simulink model "export_example"  (Simulink 8.0)
settings: Solver=ode45  StartTime=0.0  StopTime=10.0  RelTol=1e-3
libraries: aerolibactuator x1
settings Model: Creator=Marci  LastModifiedBy=Marci
settings ConfigurationSet: Description=SimMechanics 2G

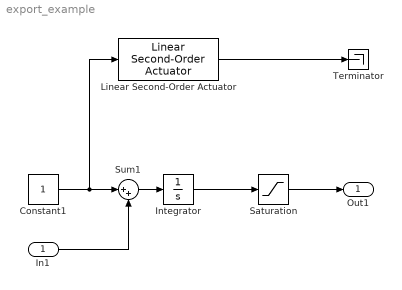
== system export_example ==
  In1 : Inport
  Constant1 : Constant
  Integrator : Integrator
  Linear Second-Order Actuator : aerolibactuator/Linear Second-Order Actuator  wn_fin=1  z_fin=0.3  fin_act_0=0  fin_act_vel=0
  Saturation : Saturate  UpperLimit=5  LowerLimit=0
  Sum1 : Sum  Inputs=|++
  Terminator : Terminator
  Out1 : Outport
  wires:
  Integrator/1 -> Saturation/1
  Saturation/1 -> Out1/1
  Sum1/1 -> Integrator/1
  Constant1/1 -> Linear Second-Order Actuator/1, Sum1/1
  In1/1 -> Sum1/2
  Linear Second-Order Actuator/1 -> Terminator/1
